simulink model "Integrated Protection, FLISR Automation, and Performance Analytics of a Smart Distribution"  (R2025b)
settings: Solver=VariableStepAuto  StartTime=0.0  StopTime=0.3  RelTol=1e-3
libraries: spsThreePhaseVIMeasurementLib x3, spsThreePhaseSourceLib x2, spsPower3phInstantaneousLib x2, spsThreePhaseBreakerLib x2, dspstat3 x1, spsRMSLib x1, simulink_extras x1, spsThreePhasePISectionLineLib x1, spsThreePhaseSeriesRLCLoadLib x1, spsThreePhaseFaultLib x1, spspowerguiLib x1
settings Model: Creator=harsh  LastModifiedBy=harsh

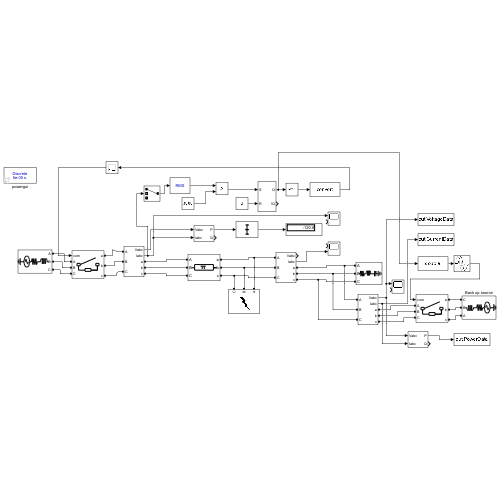
[thumbnail: Simulink's stored preview of the top-level diagram]
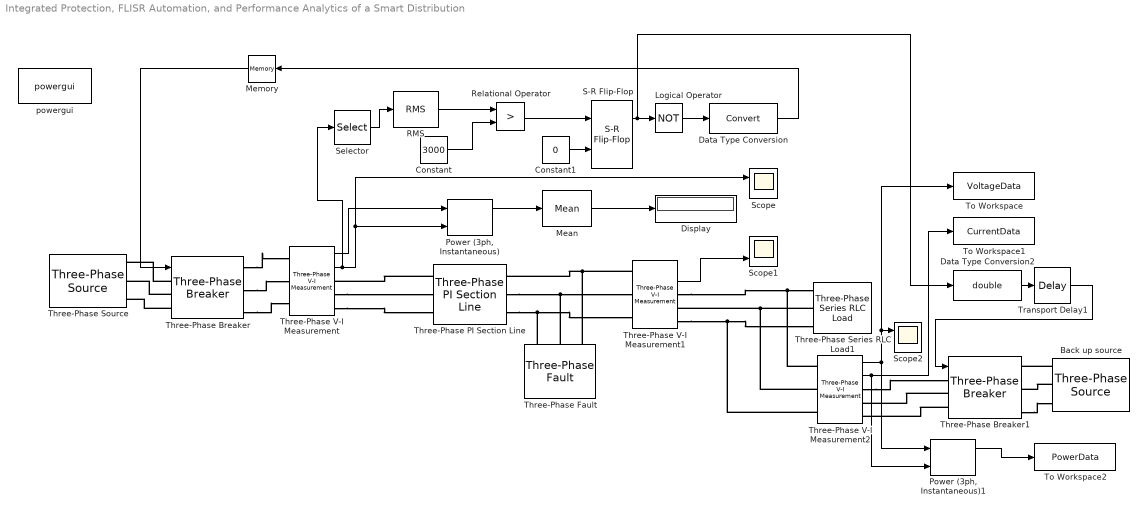
== system Integrated Protection, FLISR Automation, and Performance Analytics of a Smart Distribution ==
  Back up source : spsThreePhaseSourceLib/Three-Phase Source  InternalConnection=Yg  VoltagePhases=off  Voltage=11000  PhaseAngle=-30  Voltage_phases=[25e3 25e3 25e3]/sqrt(3)  PhaseAngles_phases=[0 -120 +120]  Frequency=50  NonIdealSource=on  SpecifyImpedance=off  Resistance=0.1  Inductance=1e-5  ShortCircuitLevel=100e6  BaseVoltage=25e3  XRratio=7  BusType=swing  Pref=10e3  Qref=0  Prefabc=[10e3, 10e3, 10e3]  Qrefabc=[0, 0, 0]  Qmin=-inf  Qmax=inf
  Constant : Constant  Value=3000  OutDataTypeStr=boolean
  Constant1 : Constant  Value=0  OutDataTypeStr=boolean
  Data Type Conversion : DataTypeConversion  SaturateOnIntegerOverflow=off  RndMeth=Floor
  Data Type Conversion2 : DataTypeConversion  OutDataTypeStr=double  SaturateOnIntegerOverflow=off  RndMeth=Floor
  Display : Display
  Logical Operator : Logic  Operator=NOT  AllPortsSameDT=off  OutDataTypeStr=boolean
  Mean : dspstat3/Mean  run=off  InputProcessing=Columns as channels (frame based)  reset_popup=None  directionMode=Each column  dimension=1  roiEnable=off  roiType=Rectangles  roiPortion=Entire ROI  roiOutput=Individual statistics for each ROI  roiFlag=off  roundingMode=Floor  overflowMode=off  outputDataTypeStr=Inherit: Same as accumulator  outputMin=[]  outputMax=[]  outputLastDataTypeStr=Inherit: Same as accumulator
  Memory : Memory  InitialCondition=1  InheritSampleTime=on
  "Power (3ph, Instantaneous)" : spsPower3phInstantaneousLib/Power (3ph, Instantaneous)
  "Power (3ph, Instantaneous)1" : spsPower3phInstantaneousLib/Power (3ph, Instantaneous)
  RMS : spsRMSLib/RMS  TrueRMS=on  Freq=50  RMSInit=0  Ts=0
  Relational Operator : RelationalOperator  Operator=>  OutDataTypeStr=boolean  RndMeth=Simplest  InputSameDT=off
  S-R Flip-Flop : simulink_extras/Flip Flops/S-R Flip-Flop  initial_condition=0
  Scope : Scope  NumInputPorts=2
      settings: ActiveDisplayYMinimum=-2717.0319391241596  ActiveDisplayYMaximum=4745.122027242116
  Scope1 : Scope  NumInputPorts=2
      settings: ActiveDisplayYMinimum=-13857.237480854366  ActiveDisplayYMaximum=15920.653439832142
  Scope2 : Scope  NumInputPorts=2
      settings: ActiveDisplayYMinimum=-10803.048565189869  ActiveDisplayYMaximum=11630.858666215045  DataLoggingVariableName=ScopeData2
  Selector : Selector  InputPortWidth=3  IndexOptions=Index vector (dialog)  Indices=[1]  OutputSizes=1
  Three-Phase PI Section Line : spsThreePhasePISectionLineLib/Three-Phase PI Section Line  LConnTagsString=a|b|c  RConnTagsString=A|B|C  Length=5  Frequency=50  Resistances=[ 0.25 0.75]  Inductances=[ 1e-3 3e-3]  Capacitances=[12.74e-9 7.75e-9]
  Three-Phase Series RLC Load1 : spsThreePhaseSeriesRLCLoadLib/Three-Phase Series RLC Load  LConnTagsString=A|B|C  Configuration=Y (grounded)  NominalVoltage=11000  Vabc=[1e3 1e3 1e3]  Vabcp=[1e3 1e3 1e3]  NominalFrequency=50  UnbalancedPower=off  ActivePower=1e6  InductivePower=100  CapacitivePower=100  Pabc=[10e3 9e3 11e3]  QLabc=[100 90 110]  QCabc=[100 90 110]  Pabcp=[10e3 9e3 11e3]  QLabcp=[100 90 110]  QCabcp=[100 90 110]  Measurements=None  LoadType=constant Z
  Three-Phase V-I Measurement : spsThreePhaseVIMeasurementLib/Three-Phase V-I Measurement  VoltageMeasurement=phase-to-ground  SetLabelV=off  LabelV=Vabc  Vpu=off  VpuLL=off  CurrentMeasurement=yes  SetLabelI=off  LabelI=Iabc  Ipu=off  Pbase=100e6  Vbase=500e3  OutputType=Complex  PhasorSimulation=off  PSBequivalent=0
  Three-Phase V-I Measurement1 : spsThreePhaseVIMeasurementLib/Three-Phase V-I Measurement  VoltageMeasurement=phase-to-ground  SetLabelV=off  LabelV=Vabc  Vpu=off  VpuLL=off  CurrentMeasurement=yes  SetLabelI=off  LabelI=Iabc  Ipu=off  Pbase=100e6  Vbase=500e3  OutputType=Complex  PhasorSimulation=off  PSBequivalent=0
  Three-Phase V-I Measurement2 : spsThreePhaseVIMeasurementLib/Three-Phase V-I Measurement  VoltageMeasurement=phase-to-ground  SetLabelV=off  LabelV=Vabc  Vpu=off  VpuLL=off  CurrentMeasurement=yes  SetLabelI=off  LabelI=Iabc  Ipu=off  Pbase=100e6  Vbase=500e3  OutputType=Complex  PhasorSimulation=off  PSBequivalent=0
  Three-Phase Breaker : spsThreePhaseBreakerLib/Three-Phase Breaker  InitialState=open  SwitchA=on  SwitchB=on  SwitchC=on  SwitchTimes="[1/60  5/60]"  External=on  BreakerResistance=0.01  SnubberResistance=1e6  SnubberCapacitance=inf  Measurements=None
  Three-Phase Breaker1 : spsThreePhaseBreakerLib/Three-Phase Breaker  InitialState=open  SwitchA=on  SwitchB=on  SwitchC=on  SwitchTimes="[1/60  5/60]"  External=on  BreakerResistance=0.01  SnubberResistance=1e6  SnubberCapacitance=inf  Measurements=None
  Three-Phase Fault : spsThreePhaseFaultLib/Three-Phase Fault  InitialStates=0  FaultA=on  FaultB=off  FaultC=off  GroundFault=on  SwitchTimes="[0.04  0.1]"  External=off  SwitchStatus=NaN  FaultResistance=0.001  GroundResistance=0.01  SnubberResistance=1e6  SnubberCapacitance=inf  Measurements=None
  Three-Phase Source : spsThreePhaseSourceLib/Three-Phase Source  InternalConnection=Yg  VoltagePhases=off  Voltage=11000  PhaseAngle=0  Voltage_phases=[25e3 25e3 25e3]/sqrt(3)  PhaseAngles_phases=[0 -120 +120]  Frequency=50  NonIdealSource=on  SpecifyImpedance=off  Resistance=0.01  Inductance=1e-5  ShortCircuitLevel=100e6  BaseVoltage=25e3  XRratio=7  BusType=swing  Pref=10e3  Qref=0  Prefabc=[10e3, 10e3, 10e3]  Qrefabc=[0, 0, 0]  Qmin=-inf  Qmax=inf
  To Workspace : ToWorkspace  VariableName=VoltageData  SampleTime=-1
  To Workspace1 : ToWorkspace  VariableName=CurrentData  SampleTime=-1
  To Workspace2 : ToWorkspace  VariableName=PowerData  SampleTime=-1
  Transport Delay1 : TransportDelay  DelayTime=0.1
  powergui : spspowerguiLib/powergui  Priority=1  SimulationMode=Discrete  SampleTime=50e-6  frequency=60  Iterations=50  frequencyindice=50  Pbase=100e6  ErrMax=1e-4  UnitsV=kV  UnitsW=MW  buscounter=0  FunctionMessages=off  echomessages=off  EnableUseOfTLC=off  CurrentSourceSwitches=off  DisableSnubberDevices=off  DisableRonSwitches=off  DisableVfSwitches=off  DisplayEquations=off  AutomaticDiscreteSolvers=off  SolverType=Tustin/Backward Euler (TBE)  Interpol=off  ExternalGateDelay=off  methode=off  Ts=100  x0status=blocks  SPID=on  SwTol=0  HookPort=off  NonlinearTolerance=1e-4  nMaxIteration=100  ContinueOnMaxIteration=off  RestoreLinks=warning  ResistiveCurrentMeasurement=off  Frange=[0:2:500]  Ylog=off  Xlog=on  ShowGrid=off  save=off  variable=ZData  structure=0  ZoomFFT=off  StartTime=0.0  cycles=1  DisplayStyle=1  fundamental=60  FreqAxis=off  MaxFrequency=1000  frequencyindicesteady=1  RmsSteady=1  display=off
  wires:
  Three-Phase V-I Measurement/1 -> "Power (3ph, Instantaneous)"/1
  Three-Phase V-I Measurement/2 -> Selector/1, Scope/1, "Power (3ph, Instantaneous)"/2
  "Power (3ph, Instantaneous)"/1 -> Mean/1
  Mean/1 -> Display/1
  Three-Phase V-I Measurement1/2 -> Scope1/2
  RMS/1 -> Relational Operator/1
  Constant/1 -> Relational Operator/2
  Relational Operator/1 -> S-R Flip-Flop/1
  Constant1/1 -> S-R Flip-Flop/2
  S-R Flip-Flop/1 -> Data Type Conversion2/1, Logical Operator/1
  Logical Operator/1 -> Data Type Conversion/1
  Selector/1 -> RMS/1
  Data Type Conversion/1 -> Memory/1
  Memory/1 -> Three-Phase Breaker/1
  Transport Delay1/1 -> Three-Phase Breaker1/1
  Three-Phase V-I Measurement2/1 -> To Workspace/1, Scope2/1, "Power (3ph, Instantaneous)1"/1
  Data Type Conversion2/1 -> Transport Delay1/1
  Three-Phase V-I Measurement2/2 -> "Power (3ph, Instantaneous)1"/2, To Workspace1/1
  "Power (3ph, Instantaneous)1"/1 -> To Workspace2/1
  connections:
  Three-Phase PI Section Line/LConn1 -- Three-Phase V-I Measurement/RConn1
  Three-Phase V-I Measurement/RConn2 -- Three-Phase PI Section Line/LConn2
  Three-Phase V-I Measurement/RConn3 -- Three-Phase PI Section Line/LConn3
  Three-Phase V-I Measurement1/LConn1 -- Three-Phase PI Section Line/RConn1 -- Three-Phase Fault/LConn1
  Three-Phase PI Section Line/RConn2 -- Three-Phase Fault/LConn2 -- Three-Phase V-I Measurement1/LConn2
  Three-Phase PI Section Line/RConn3 -- Three-Phase Fault/LConn3 -- Three-Phase V-I Measurement1/LConn3
  Three-Phase Series RLC Load1/LConn2 -- Three-Phase V-I Measurement2/LConn2 -- Three-Phase V-I Measurement1/RConn2
  Three-Phase V-I Measurement1/RConn1 -- Three-Phase V-I Measurement2/LConn1 -- Three-Phase Series RLC Load1/LConn1
  Three-Phase V-I Measurement1/RConn3 -- Three-Phase V-I Measurement2/LConn3 -- Three-Phase Series RLC Load1/LConn3
  Three-Phase Breaker/LConn1 -- Three-Phase Source/RConn1
  Three-Phase Breaker/LConn2 -- Three-Phase Source/RConn2
  Three-Phase Breaker/LConn3 -- Three-Phase Source/RConn3
  Three-Phase Breaker/RConn2 -- Three-Phase V-I Measurement/LConn2
  Three-Phase Breaker/RConn1 -- Three-Phase V-I Measurement/LConn1
  Three-Phase Breaker/RConn3 -- Three-Phase V-I Measurement/LConn3
  Back up source/RConn2 -- Three-Phase Breaker1/RConn2
  Back up source/RConn3 -- Three-Phase Breaker1/RConn1
  Three-Phase Breaker1/RConn3 -- Back up source/RConn1
  Three-Phase V-I Measurement2/RConn1 -- Three-Phase Breaker1/LConn1
  Three-Phase Breaker1/LConn2 -- Three-Phase V-I Measurement2/RConn2
  Three-Phase Breaker1/LConn3 -- Three-Phase V-I Measurement2/RConn3
